simulink model "laserESClazoCerrado"  (R2021a)
settings: Solver=FixedStepDiscrete  StartTime=0.0  StopTime=tSim  FixedStep=tSamp  MaxStep=tSamp  RelTol=1e-9  EnableMultiTasking=on
values from neighbouring files (symbols this model uses):
  Aesc = 0.12    [simulacionLazoCerrado.m]
  Ci = -22.5    [simulacionLazoCerrado.m]
  Cpzt = 33    [simulacionLazoCerrado.m]
  fmod = 140    [simulacionLazoCerrado.m]
  I = 300    [simulacionLazoCerrado.m]
  nCut = round(tauLock*fSamp)    [simulacionLazoCerrado.m]
  Nu0R = 10    [simulacionLazoCerrado.m]
  P = 5    [simulacionLazoCerrado.m]
  paramIntegral = ones(1,nCut)    [simulacionLazoCerrado.m]
  Slock = 1500    [simulacionLazoCerrado.m]
  tDAQ = 1200*tSamp    (= 0.184615384615)    [simulacionLazoCerrado.m]
  tInitPID = 5    [simulacionLazoCerrado.m]
  tSamp = 1/fSamp    (= 0.000153846153846)    [simulacionLazoCerrado.m]
undefined symbols (not defined in the file or in its folder): DiscIntNeverNeededParam, gaussian, nuScan, Vpd
libraries: simulink x4, eeGeneralControl x2, pid_lib x1
settings Model: Creator=Nicolas  LastModifiedBy=Nicolas
settings SolverCC: AlgebraicLoopSolver=LineSearch  ODENIntegrationMethod=ode4
settings DebuggingCC: SFMachineParentedDataDiag=warning

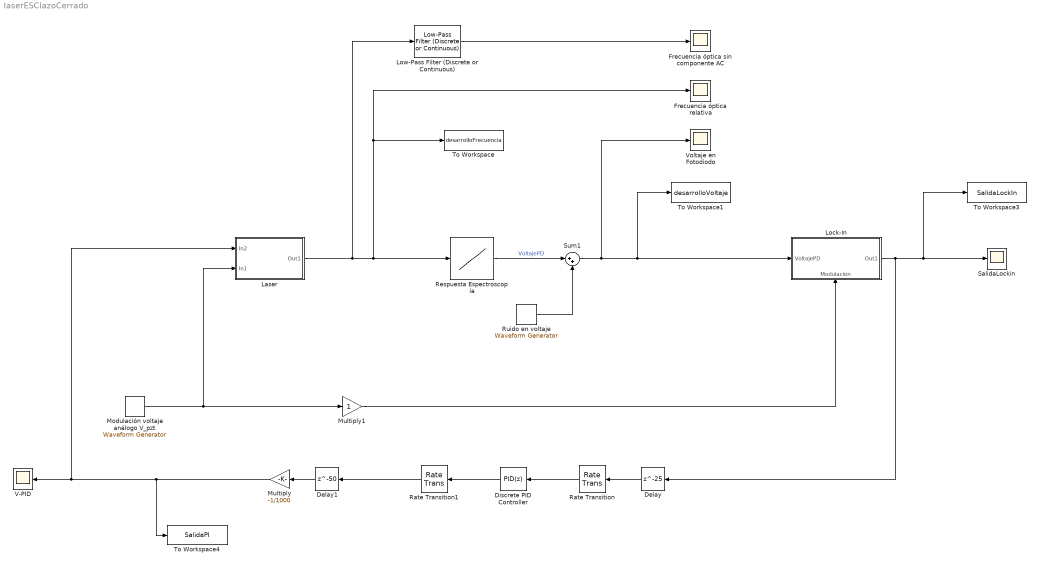
== system laserESClazoCerrado ==
  Delay : Delay  DelayLength=25
  Delay1 : Delay  DelayLength=50
  Discrete PID Controller : pid_lib/PID Controller  Controller=PID  Form=Parallel  TimeDomain=Discrete-time  UseExternalTs=off  SampleTime=tDAQ  IntegratorMethod=Forward Euler  FilterMethod=Forward Euler  ControllerParametersSource=internal  P=P  I=5*I  D=0  UseFilter=off  N=100  TunerSelectOption=Frequency Response Based  InitialConditionSource=internal  InitialConditionForIntegrator=0  InitialConditionForFilter=0  DifferentiatorICPrevScaledInput=0  ExternalReset=none  TrackingMode=off  Kt=1  LimitOutput=off  SatLimitsSource=internal  UpperSaturationLimit=inf  LowerSaturationLimit=-inf  LinearizeAsGain=off  AntiWindupMode=none  Kb=1  POutMin=[]  POutMax=[]  IOutMin=[]  IOutMax=[]  DOutMin=[]  DOutMax=[]  NOutMin=[]  NOutMax=[]  SumOutMin=[]  SumOutMax=[]  SaturationOutMin=[]  SaturationOutMax=[]  PParamMin=[]  PParamMax=[]  IParamMin=[]  IParamMax=[]  DParamMin=[]  DParamMax=[]  NParamMin=[]  NParamMax=[]  KbParamMin=[]  KbParamMax=[]  KtParamMin=[]  KtParamMax=[]  KbOutMin=[]  KbOutMax=[]  KtOutMin=[]  KtOutMax=[]  IntegratorOutMin=[]  IntegratorOutMax=[]  FilterOutMin=[]  FilterOutMax=[]  SumI1OutMin=[]  SumI1OutMax=[]  SumI2OutMin=[]  SumI2OutMax=[]  SumI3OutMin=[]  SumI3OutMax=[]  SumI4OutMin=[]  SumI4OutMax=[]  SumDOutMin=[]  SumDOutMax=[]  DifferentiatorOutMin=[]  DifferentiatorOutMax=[]  FilterDiffOutCoefMin=[]  FilterDiffOutCoefMax=[]  ReciprocalOutMin=[]  ReciprocalOutMax=[]  SumDenOutMin=[]  SumDenOutMax=[]  SumNumOutMin=[]  SumNumOutMax=[]  DivideOutMin=[]  DivideOutMax=[]  UdiffTsProdOutMin=[]  UdiffTsProdOutMax=[]  NTsProdOutMin=[]  NTsProdOutMax=[]  UintegralTsProdOutMin=[]  UintegralTsProdOutMax=[]  UngainTsProdOutMin=[]  UngainTsProdOutMax=[]  IntegratorContinuousStateAttributes=''  IntegratorStateMustResolveToSignalObject=off  IntegratorRTWStateStorageClass=Auto  FilterContinuousStateAttributes=''  FilterStateMustResolveToSignalObject=off  FilterRTWStateStorageClass=Auto  ParallelPVariant=InternalParameters  IdealPVariant=Disabled  IVariant=InternalParameters  DVariant=InternalParameters  IntegratorVariant=Discrete  SatVariant=Disabled  AWVariant=Passthrough  PCopyVariant=Disabled  TRVariant=Disabled  FdbkBlocksVariant=Forward  IdealPFdbkVariant=Disabled  SatFdbkVariant=Disabled  DerivativeFilterVariant=Differentiator  NVariant=Passthrough  NCopyVariant=Disabled_SignalSpec  FilterICVariant=InternalICsDifferentiator  IntegratorICVariant=InternalICs  ExternalResetVariant=Disabled  TRSumVariant=Passthrough  SumFdbkVariant=Disabled  SumVariant=Sum_PID  TsampFilterVariant=InternalTs  TsampNgainVariant=Passthrough  TsampIntegralVariant=Passthrough  ExternalSaturationOutDataTypeStr=Inherit: Same as second input
  Frecuencia óptica relativa : Scope
  Frecuencia óptica sin componente AC : Scope
  Laser : Subsystem
  Lock-In : Subsystem
      settings: PortSchema="{\"entries\":[{\"content\":{\"sides\":[{\"content\":{\"connectorIds\":[\"In1\"]},\"type\":\"ConnectorPlacement.EquallySpacedRectSide\",\"uuid\":\"22eb7a48-a65d-4f64-b6ee-dff5559d7a34\"},{\"content\":{\"connectorIds\":[\"Out1\"],\"side\":\"RIGHT\"},\"type\":\"ConnectorPlacement.EquallySpacedRectSide\",\"uuid\":\"cbb02784-070d-4c05-96b0-2cd4d8e414fc\"},{\"content\":{\"connectorIds\":[],\"side\":\"TOP\"},\"type\":\"ConnectorPlacement.EquallySpacedRectSide\",\"uuid\":\"e508e192-dcc2-4bb3-9075-558ee8a381ef\"},{\"content\":{\"connectorIds\":[\"In2\"],\"side\":\"BOTTOM\"},\"type\":\"ConnectorPlacement.EquallySpacedRectSide\",\"uuid\":\"019199a6-8006-4a7e-aaa3-3e961b2e19ac\"}]},\"type\":\"ConnectorPlacement.EquallySpacedConnector\",\"uuid\":\"b458a542-b98a-4352-bbf7-718e0f3341fd\"}],\"packageUris\":[\"http://schema.mathworks.com/mf0/Connector/19700101\"],\"version\":\"1.0\"}"
  Low-Pass Filter (Discrete or Continuous) : eeGeneralControl/Low-Pass Filter (Discrete or Continuous)  K=1  T=10/fmod  B=inf  A=-inf  init_option=Inherited from block input  x0=0  Ts=-1
  Modulación voltaje análogo V_pzt : simulink/Sources/Waveform Generator  OutMin=[]  OutMax=[]  OutDataTypeStr=double  SelectedSignal=1  Signals=sin('Amplitude',Aesc,'Frequency',fmod*2*pi,'Phase',0)  BlockNames=MultiportSwitch_a689d72bae7f4a1  SampleTime=tSamp
  Multiply : Gain  Gain=-1/1000
  Multiply1 : Gain
  Rate Transition : RateTransition  OutPortSampleTimeOpt=Inherit
  Rate Transition1 : RateTransition  OutPortSampleTimeOpt=Inherit
  Respuesta Espectroscopía : Lookup_n-D  NumberOfTableDimensions=1  BreakpointsForDimension1=nuScan  Table=Vpd  InterpMethod=Nearest  RndMeth=Simplest  InputSameDT=on
  Ruido en voltaje : simulink/Sources/Waveform Generator  OutMin=[]  OutMax=[]  OutDataTypeStr=double  SelectedSignal=1  Signals=gaussian(0,0.000075,0)  BlockNames=MultiportSwitch_6b159e8dbbe44bb  SampleTime=tSamp
  SalidaLockin : Scope
  Sum1 : Sum  Inputs=|++
  To Workspace : ToWorkspace  VariableName=desarrolloFrecuencia  SaveFormat=Timeseries  SampleTime=-1
  To Workspace1 : ToWorkspace  VariableName=desarrolloVoltaje  SaveFormat=Timeseries  SampleTime=-1
  To Workspace3 : ToWorkspace  VariableName=SalidaLockIn  SaveFormat=Timeseries  SampleTime=-1
  To Workspace4 : ToWorkspace  VariableName=SalidaPI  SaveFormat=Timeseries  SampleTime=-1
  V-PID : Scope
  Voltaje en Fotodiodo : Scope
  wires:
  Low-Pass Filter (Discrete or Continuous)/1 -> Frecuencia óptica sin componente AC/1
  Laser/1(Out1) -> To Workspace/1, Frecuencia óptica relativa/1, Respuesta Espectroscopía/1, Low-Pass Filter (Discrete or Continuous)/1
  Lock-In/1(Out1) -> To Workspace3/1, SalidaLockin/1, Delay/1
  Modulación voltaje análogo V_pzt/1 -> Laser/2(In1), Multiply1/1
  Ruido en voltaje/1 -> Sum1/2
  Respuesta Espectroscopía/1 -> Sum1/1  "VoltajePD"
  Sum1/1 -> Voltaje en Fotodiodo/1, Lock-In/1(VoltajePD), To Workspace1/1
  Multiply1/1 -> Lock-In/2(Modulacion)
  Delay/1 -> Rate Transition/1
  Discrete PID Controller/1 -> Rate Transition1/1
  Rate Transition/1 -> Discrete PID Controller/1
  Rate Transition1/1 -> Delay1/1
  Delay1/1 -> Multiply/1
  Multiply/1 -> To Workspace4/1, Laser/1(In2), V-PID/1

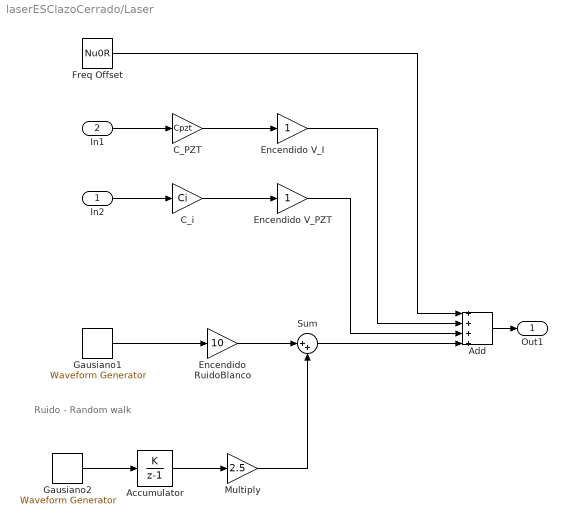
== system laserESClazoCerrado/Laser ==
  note: Ruido - Random walk
  In2 : Inport
  In1 : Inport  Port=2
  Accumulator : DiscreteIntegrator  IntegratorMethod=Accumulation: Forward Euler  SampleTime=-1  ICPrevOutput=DiscIntNeverNeededParam  ICPrevScaledInput=DiscIntNeverNeededParam
  Add : Sum  Inputs=++++
  C_PZT : Gain  Gain=Cpzt
  C_i : Gain  Gain=Ci
  Encendido RuidoBlanco : Gain  Gain=10
  Encendido V_I : Gain
  Encendido V_PZT : Gain
  Freq Offset : Constant  Value=Nu0R
  Gausiano1 : simulink/Sources/Waveform Generator  OutMin=[]  OutMax=[]  OutDataTypeStr=double  SelectedSignal=1  Signals=gaussian(0,0.1,0)  BlockNames=MultiportSwitch_9bbf6bd2c6724f1  SampleTime=tSamp
  Gausiano2 : simulink/Sources/Waveform Generator  OutMin=[]  OutMax=[]  OutDataTypeStr=double  SelectedSignal=1  Signals=gaussian(0,1e-4,0)  BlockNames=MultiportSwitch_e088cc4a76fd441  SampleTime=tSamp
  Multiply : Gain  Gain=2.5
  Sum : Sum  Inputs=|++
  Out1 : Outport
  wires:
  Add/1 -> Out1/1
  Gausiano2/1 -> Accumulator/1
  Freq Offset/1 -> Add/1
  In1/1 -> C_PZT/1
  C_PZT/1 -> Encendido V_I/1
  C_i/1 -> Encendido V_PZT/1
  Accumulator/1 -> Multiply/1
  In2/1 -> C_i/1
  Sum/1 -> Add/4
  Gausiano1/1 -> Encendido RuidoBlanco/1
  Multiply/1 -> Sum/2
  Encendido V_I/1 -> Add/2
  Encendido V_PZT/1 -> Add/3
  Encendido RuidoBlanco/1 -> Sum/1

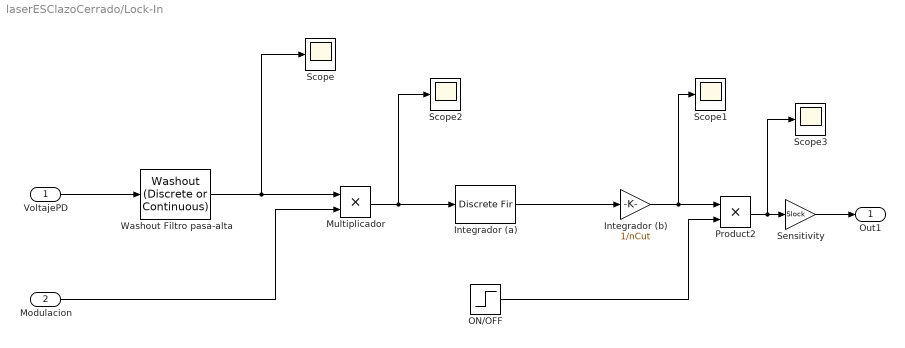
== system laserESClazoCerrado/Lock-In ==
  VoltajePD : Inport
  Modulacion : Inport  Port=2
  Integrador (a) : DiscreteFir  Coefficients=paramIntegral
  Integrador (b) : Gain  Gain=1/nCut
  Multiplicador : Product
  ON/OFF : Step  Time=tInitPID
  Product2 : Product
  Scope{,1..3} (4 alike) : Scope
  Sensitivity : Gain  Gain=Slock
  Washout Filtro pasa-alta : eeGeneralControl/Washout (Discrete or Continuous)  T=1/(fmod*0.95)  init_option=Inherited from block input  x0=0  Ts=-1
      settings: SourceProductBaseCode=PS
  Out1 : Outport
  wires:
  Modulacion/1 -> Multiplicador/2
  Washout Filtro pasa-alta/1 -> Scope/1, Multiplicador/1
  Integrador (a)/1 -> Integrador (b)/1
  Integrador (b)/1 -> Scope1/1, Product2/1
  Product2/1 -> Scope3/1, Sensitivity/1
  ON/OFF/1 -> Product2/2
  Multiplicador/1 -> Scope2/1, Integrador (a)/1
  VoltajePD/1 -> Washout Filtro pasa-alta/1
  Sensitivity/1 -> Out1/1
